simulink model "DifferentialDrivePIDModel"  (R2020b)
settings: Solver=VariableStepAuto  StartTime=0.0  StopTime=20  RelTol=1e-3
undefined symbols (not defined in the file): L, limit_vel, r
libraries: simulink_extras x2, simulink x1
settings Model: Creator=USER  LastModifiedBy=USER

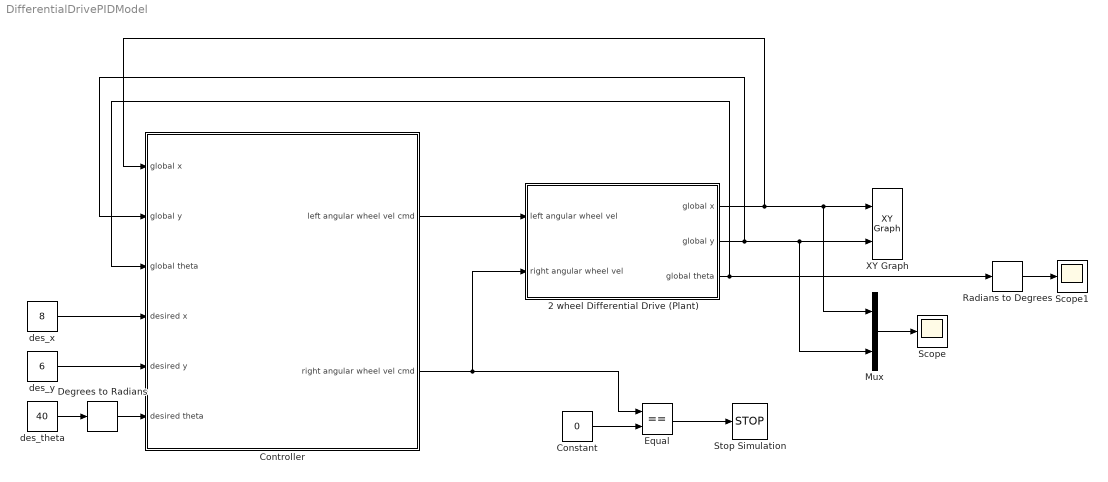
== system DifferentialDrivePIDModel ==
  2 wheel Differential Drive (Plant) : Subsystem
  Constant : Constant  Value=0
  Controller : Subsystem
  Degrees to Radians : simulink_extras/Transformations/Degrees to Radians
  Equal : RelationalOperator  Operator===  OutDataTypeStr=boolean  ZeroCross=off  RndMeth=Zero
  Mux : Mux  Inputs=2
  Radians to Degrees : simulink_extras/Transformations/Radians to Degrees
  Scope : Scope
  Scope1 : Scope
  Stop Simulation : Stop
  XY Graph : simulink/Sinks/XY Graph  xmin=-1  xmax=10  ymin=-1  ymax=10  st=-1
  des_theta : Constant  Value=40
  des_x : Constant  Value=8
  des_y : Constant  Value=6
  wires:
  Controller/1(left angular wheel vel cmd) -> 2 wheel Differential Drive (Plant)/1(left angular wheel vel)
  Controller/2(right angular wheel vel cmd) -> Equal/1, 2 wheel Differential Drive (Plant)/2(right angular wheel vel)
  2 wheel Differential Drive (Plant)/1(global x) -> Mux/1, XY Graph/1, Controller/1(global x)
  2 wheel Differential Drive (Plant)/2(global y) -> Mux/2, XY Graph/2, Controller/2(global y)
  2 wheel Differential Drive (Plant)/3(global theta) -> Radians to Degrees/1, Controller/3(global theta)
  des_x/1 -> Controller/4(desired x)
  des_theta/1 -> Degrees to Radians/1
  des_y/1 -> Controller/5(desired y)
  Equal/1 -> Stop Simulation/1
  Constant/1 -> Equal/2
  Mux/1 -> Scope/1
  Radians to Degrees/1 -> Scope1/1
  Degrees to Radians/1 -> Controller/6(desired theta)

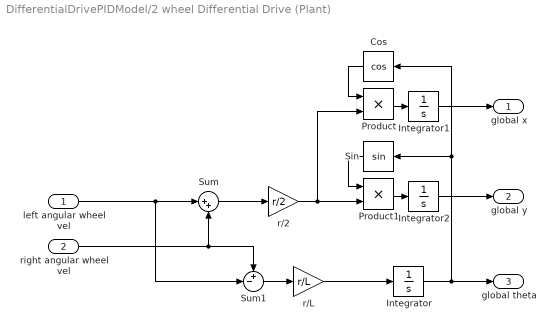
== system DifferentialDrivePIDModel/2 wheel Differential Drive (Plant) ==
  left angular wheel vel : Inport
  right angular wheel vel : Inport  Port=2
  Cos : Trigonometry  Operator=cos
  Integrator : Integrator
  Integrator1 : Integrator
  Integrator2 : Integrator
  Product : Product
  Product1 : Product
  Sin : Trigonometry
  Sum : Sum  Inputs=|++
  Sum1 : Sum  Inputs=+-|
  r/2 : Gain  Gain=r/2
  r/L : Gain  Gain=r/L
  global x : Outport
  global y : Outport  Port=2
  global theta : Outport  Port=3
  wires:
  left angular wheel vel/1 -> Sum1/2, Sum/1
  right angular wheel vel/1 -> Sum1/1, Sum/2
  Sum/1 -> r/2/1
  Sum1/1 -> r/L/1
  r/L/1 -> Integrator/1
  Integrator/1 -> Cos/1, Sin/1, global theta/1
  Cos/1 -> Product/1
  Sin/1 -> Product1/1
  r/2/1 -> Product/2, Product1/2
  Product/1 -> Integrator1/1
  Integrator1/1 -> global x/1
  Product1/1 -> Integrator2/1
  Integrator2/1 -> global y/1

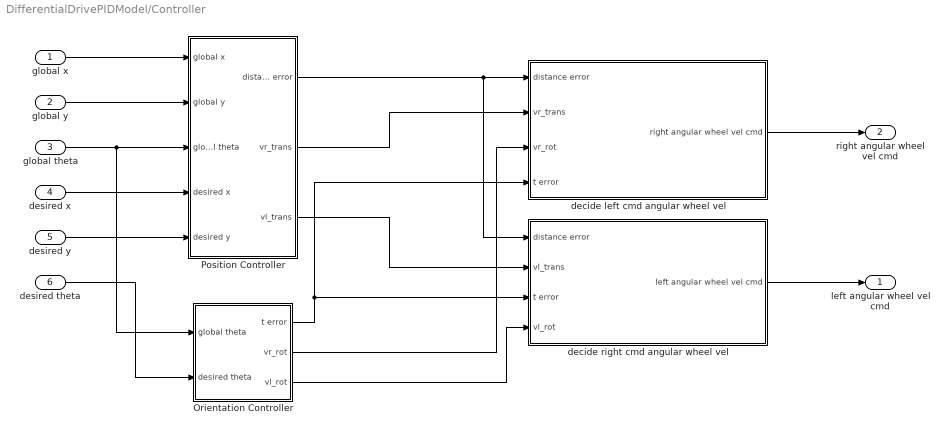
== system DifferentialDrivePIDModel/Controller ==
  global x : Inport
  global y : Inport  Port=2
  global theta : Inport  Port=3
  desired x : Inport  Port=4
  desired y : Inport  Port=5
  desired theta : Inport  Port=6
  Orientation Controller : Subsystem
  Position Controller : Subsystem
  decide left cmd angular wheel vel : Subsystem
  decide right cmd angular wheel vel : Subsystem
  left angular wheel vel cmd : Outport
  right angular wheel vel cmd : Outport  Port=2
  wires:
  global x/1 -> Position Controller/1(global x)
  global y/1 -> Position Controller/2(global y)
  global theta/1 -> Orientation Controller/1(global theta), Position Controller/3(global theta)
  desired x/1 -> Position Controller/4(desired x)
  desired y/1 -> Position Controller/5(desired y)
  desired theta/1 -> Orientation Controller/2(desired theta)
  Position Controller/1(distance error) -> decide right cmd angular wheel vel/1(distance error), decide left cmd angular wheel vel/1(distance error)
  Position Controller/2(vr_trans) -> decide left cmd angular wheel vel/2(vr_trans)
  Orientation Controller/2(vr_rot) -> decide left cmd angular wheel vel/3(vr_rot)
  Orientation Controller/1(t error) -> decide left cmd angular wheel vel/4(t error), decide right cmd angular wheel vel/3(t error)
  Orientation Controller/3(vl_rot) -> decide right cmd angular wheel vel/4(vl_rot)
  Position Controller/3(vl_trans) -> decide right cmd angular wheel vel/2(vl_trans)
  decide left cmd angular wheel vel/1(right angular wheel vel cmd) -> right angular wheel vel cmd/1
  decide right cmd angular wheel vel/1(left angular wheel vel cmd) -> left angular wheel vel cmd/1

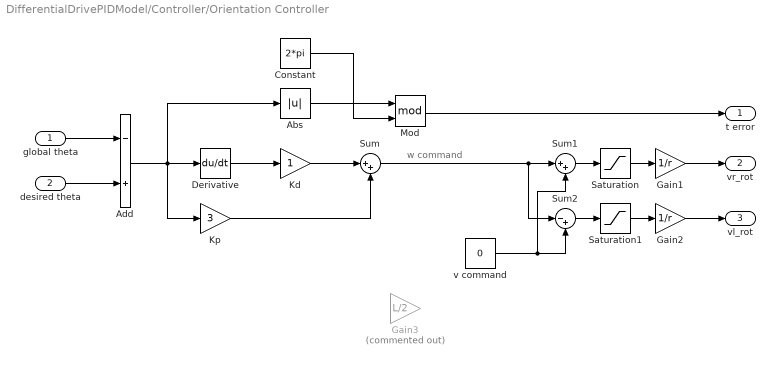
== system DifferentialDrivePIDModel/Controller/Orientation Controller ==
  note: w command
  global theta : Inport
  desired theta : Inport  Port=2
  Abs : Abs
  Add : Sum  Inputs=-+
  Constant : Constant  Value=2*pi
  Derivative : Derivative
  Gain1 : Gain  Gain=1/r
  Gain2 : Gain  Gain=1/r
  Gain3 : Gain  Commented=on  Gain=L/2
  Kd : Gain
  Kp : Gain  Gain=3
  Mod : Math  Operator=mod  SaturateOnIntegerOverflow=on
  Saturation : Saturate  UpperLimit=limit_vel  LowerLimit=-limit_vel  ZeroCross=off
  Saturation1 : Saturate  UpperLimit=limit_vel  LowerLimit=-limit_vel  ZeroCross=off
  Sum : Sum  Inputs=|++
  Sum1 : Sum  Inputs=|++
  Sum2 : Sum  Inputs=|-+
  v command : Constant  Value=0
  t error : Outport
  vr_rot : Outport  Port=2
  vl_rot : Outport  Port=3
  wires:
  global theta/1 -> Add/1
  desired theta/1 -> Add/2
  Add/1 -> Abs/1, Kp/1, Derivative/1
  Kd/1 -> Sum/1
  Kp/1 -> Sum/2
  Derivative/1 -> Kd/1
  Abs/1 -> Mod/1
  Constant/1 -> Mod/2
  Mod/1 -> t error/1
  Sum/1 -> Sum2/1, Sum1/1
  v command/1 -> Sum1/2, Sum2/2
  Sum1/1 -> Saturation/1
  Sum2/1 -> Saturation1/1
  Saturation/1 -> Gain1/1
  Saturation1/1 -> Gain2/1
  Gain1/1 -> vr_rot/1
  Gain2/1 -> vl_rot/1

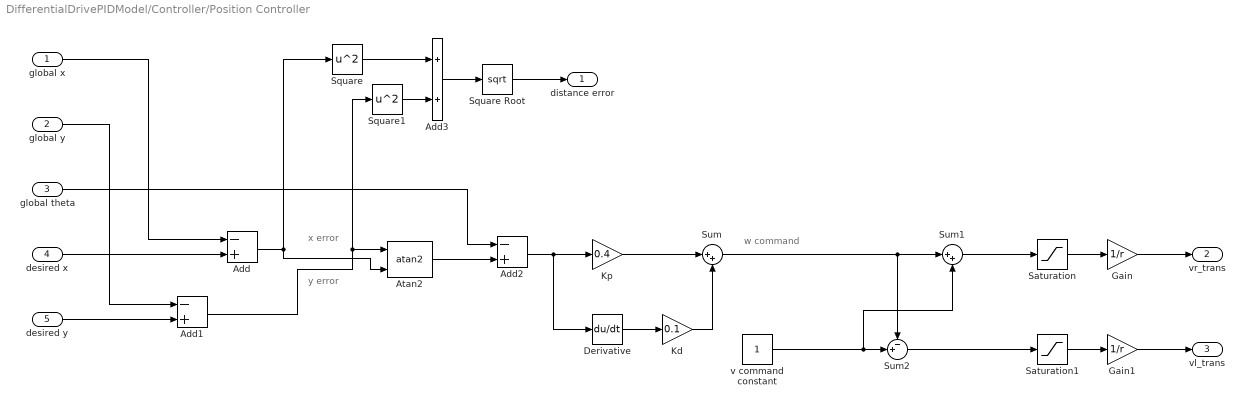
== system DifferentialDrivePIDModel/Controller/Position Controller ==
  note: x error
  note: y error
  note: w command
  global x : Inport
  global y : Inport  Port=2
  global theta : Inport  Port=3
  desired x : Inport  Port=4
  desired y : Inport  Port=5
  Add : Sum  Inputs=-+
  Add1 : Sum  Inputs=-+
  Add2 : Sum  Inputs=-+
  Add3 : Sum
  Atan2 : Trigonometry  Operator=atan2
  Derivative : Derivative
  Gain : Gain  Gain=1/r
  Gain1 : Gain  Gain=1/r
  Kd : Gain  Gain=0.1
  Kp : Gain  Gain=0.4
  Saturation : Saturate  UpperLimit=limit_vel  LowerLimit=-limit_vel  ZeroCross=off
  Saturation1 : Saturate  UpperLimit=limit_vel  LowerLimit=-limit_vel  ZeroCross=off
  Square : Math  Operator=square  SaturateOnIntegerOverflow=on
  Square Root : Sqrt  SaturateOnIntegerOverflow=on
  Square1 : Math  Operator=square  SaturateOnIntegerOverflow=on
  Sum : Sum  Inputs=|++
  Sum1 : Sum  Inputs=|++
  Sum2 : Sum  Inputs=-+|
  v command constant : Constant
  distance error : Outport
  vr_trans : Outport  Port=2
  vl_trans : Outport  Port=3
  wires:
  desired y/1 -> Add1/2
  desired x/1 -> Add/2
  global x/1 -> Add/1
  global y/1 -> Add1/1
  Add/1 -> Square/1, Atan2/2
  Add1/1 -> Atan2/1, Square1/1
  Atan2/1 -> Add2/2
  global theta/1 -> Add2/1
  Add2/1 -> Derivative/1, Kp/1
  Derivative/1 -> Kd/1
  Kp/1 -> Sum/1
  Kd/1 -> Sum/2
  Square1/1 -> Add3/2
  Square/1 -> Add3/1
  Add3/1 -> Square Root/1
  Square Root/1 -> distance error/1
  Sum1/1 -> Saturation/1
  Saturation/1 -> Gain/1
  Saturation1/1 -> Gain1/1
  Sum2/1 -> Saturation1/1
  Gain/1 -> vr_trans/1
  v command constant/1 -> Sum1/2, Sum2/2
  Sum/1 -> Sum1/1, Sum2/1
  Gain1/1 -> vl_trans/1

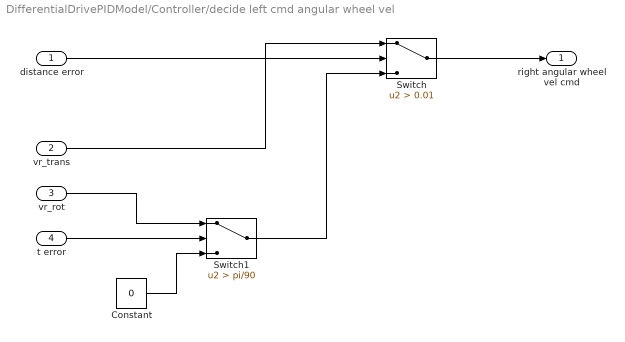
== system DifferentialDrivePIDModel/Controller/decide left cmd angular wheel vel ==
  distance error : Inport
  vr_trans : Inport  Port=2
  vr_rot : Inport  Port=3
  t error : Inport  Port=4
  Constant : Constant  Value=0
  Switch : Switch  Criteria=u2 > Threshold  Threshold=0.01
  Switch1 : Switch  Criteria=u2 > Threshold  Threshold=pi/90
  right angular wheel vel cmd : Outport
  wires:
  Switch/1 -> right angular wheel vel cmd/1
  t error/1 -> Switch1/2
  Constant/1 -> Switch1/3
  vr_rot/1 -> Switch1/1
  distance error/1 -> Switch/2
  vr_trans/1 -> Switch/1
  Switch1/1 -> Switch/3

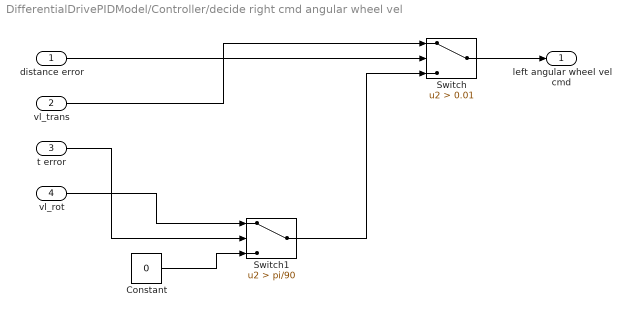
== system DifferentialDrivePIDModel/Controller/decide right cmd angular wheel vel ==
  distance error : Inport
  vl_trans : Inport  Port=2
  t error : Inport  Port=3
  vl_rot : Inport  Port=4
  Constant : Constant  Value=0
  Switch : Switch  Criteria=u2 > Threshold  Threshold=0.01
  Switch1 : Switch  Criteria=u2 > Threshold  Threshold=pi/90
  left angular wheel vel cmd : Outport
  wires:
  Constant/1 -> Switch1/3
  vl_rot/1 -> Switch1/1
  distance error/1 -> Switch/2
  t error/1 -> Switch1/2
  Switch1/1 -> Switch/3
  vl_trans/1 -> Switch/1
  Switch/1 -> left angular wheel vel cmd/1
